simulink model "factor_myfuzzy"  (R2017a)
settings: Solver=VariableStepAuto  StartTime=0.0  StopTime=10.0
undefined symbols (not defined in the file or in its folder): f1, f3
libraries: fuzblock x2
settings Model: Creator=Administrator  LastModifiedBy=Lenovo
settings SolverCC: ZeroCrossControl=DisableAll  ZeroCrossAlgorithm=Adaptive

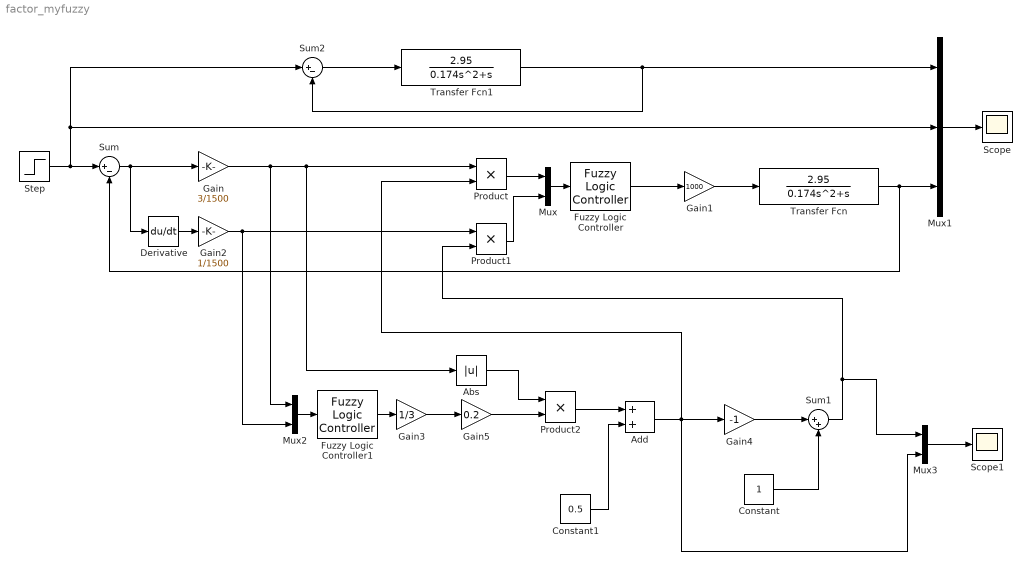
== system factor_myfuzzy ==
  Abs : Abs
  Add : Sum
  Constant : Constant
  Constant1 : Constant  Value=0.5
  Derivative : Derivative
  Fuzzy Logic Controller : fuzblock/Fuzzy Logic  Controller  fis=[f1]
  Fuzzy Logic Controller1 : fuzblock/Fuzzy Logic  Controller  fis=[f3]
  Gain : Gain  Gain=3/1500
  Gain1 : Gain  Gain=1000
  Gain2 : Gain  Gain=1/1500
  Gain3 : Gain  Gain=1/3
  Gain4 : Gain  Gain=-1
  Gain5 : Gain  Gain=0.2
  Mux : Mux  Inputs=2
  Mux1 : Mux  Inputs=3
  Mux2 : Mux  Inputs=2
  Mux3 : Mux  Inputs=2
  Product : Product
  Product1 : Product
  Product2 : Product
  Scope : Scope
  Scope1 : Scope
  Step : Step  After=1500  SampleTime=0.01
  Sum : Sum  Inputs=|+-
  Sum1 : Sum  Inputs=|++
  Sum2 : Sum  Inputs=|+-
  Transfer Fcn : TransferFcn  Numerator=[2.95]  Denominator=[0.174 1 0]
  Transfer Fcn1 : TransferFcn  Numerator=[2.95]  Denominator=[0.174 1 0]
  wires:
  Step/1 -> Mux1/2, Sum2/1, Sum/1
  Mux/1 -> Fuzzy Logic Controller/1
  Transfer Fcn/1 -> Mux1/3, Sum/2
  Transfer Fcn1/1 -> Mux1/1, Sum2/2
  Sum2/1 -> Transfer Fcn1/1
  Mux1/1 -> Scope/1
  Mux2/1 -> Fuzzy Logic Controller1/1
  Product/1 -> Mux/1
  Product1/1 -> Mux/2
  Fuzzy Logic Controller/1 -> Gain1/1
  Sum/1 -> Gain/1, Derivative/1
  Derivative/1 -> Gain2/1
  Gain/1 -> Mux2/1, Abs/1, Product/1
  Gain1/1 -> Transfer Fcn/1
  Gain2/1 -> Mux2/2, Product1/1
  Fuzzy Logic Controller1/1 -> Gain3/1
  Gain3/1 -> Gain5/1
  Gain5/1 -> Product2/2
  Abs/1 -> Product2/1
  Product2/1 -> Add/1
  Constant1/1 -> Add/2
  Add/1 -> Mux3/2, Product/2, Gain4/1
  Gain4/1 -> Sum1/1
  Constant/1 -> Sum1/2
  Sum1/1 -> Mux3/1, Product1/2
  Mux3/1 -> Scope1/1
